simulink model "VU_NXTWay"  (Simulink 10.0)
settings: Solver=FixedStepDiscrete  StartTime=0.0  StopTime=inf  FixedStep=0.004  RelTol=1e-3
PreLoadFcn:
  | param_nxtway_gs
undefined symbols (not defined in the file): a_b, a_d, a_gc, a_gd, a_r, dst_thr, gp_max, k_f, k_i, k_phidot, k_sync, k_thetadot, pwm_gain, sound_freq, time_auto, time_start, ts1, turn_angle
libraries: lego_nxt_lib x9, simulink x1
settings Model: Creator=jpeytonj  LastModifiedBy=bhisma
settings DataIOCC: LimitDataPoints=on  SignalLoggingSaveFormat=ModelDataLogs
settings OptimizationCC: ExpressionDepthLimit=2147483647
settings DebuggingCC: SolverPrmCheckMsg=warning  SingleTaskRateTransMsg=warning  FcnCallInpInsideContextMsg=warning  StateNameClashWarn=warning
settings RTWCC: Description=Lego NXT Real-Time Target  SystemTargetFile=lrt.tlc  GenCodeOnly=on  TemplateMakefile=lrt_ecrobot.tmf
settings STFCustomTargetCC: ModelReferenceCompliant=off  GeneratePreprocessorConditionals=Disable all  MatFileLogging=on  CPPClassGenCompliant=on  SystemTargetFile=lrt.tlc
settings GRTTargetCC: ModelReferenceCompliant=off  ParMdlRefBuildCompliant=off  CompOptLevelCompliant=off  ConcurrentExecutionCompliant=off  GeneratePreprocessorConditionals=Disable all  UseToolchainInfoCompliant=off  ExtModeMexFile=noextcomm
settings CustomProperty: DataType=RTWOptions_EnumType_C__LegoMindstorms_VU-LRT_lrt_1codeGenType  Value=Integer-only
settings EnumStrPairs: String=Integer-only
settings ConfigComp: CovExternalEMLEnable=off

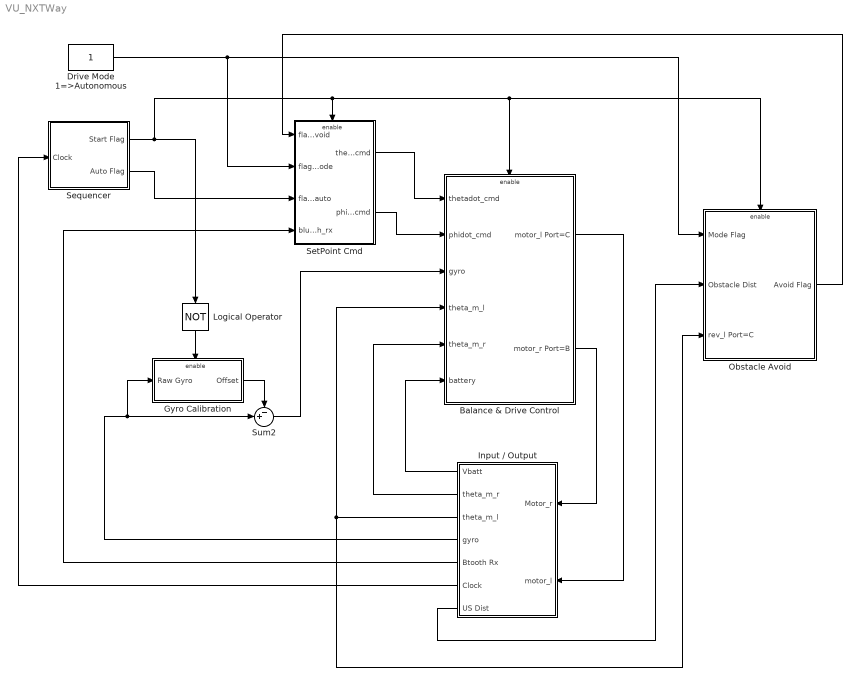
== system VU_NXTWay ==
  Balance & Drive Control : Subsystem
  Drive Mode 1=>Autonomous : Constant  OutDataTypeStr=boolean  SampleTime=-1
      settings: AttributesFormatString=DataType = %<OutDataTypeStr>
  Gyro Calibration : Subsystem  TreatAsAtomicUnit=on
  Input / Output : Subsystem
  Logical Operator : Logic  Operator=NOT  AllPortsSameDT=off  OutDataTypeStr=boolean
  Obstacle Avoid : Subsystem
  Sequencer : Subsystem
  SetPoint Cmd : Subsystem
  Sum2 : Sum  Inputs=-+|  OutDataTypeStr=Inherit: Same as first input
  wires:
  Input / Output/4(gyro) -> Gyro Calibration/1(Raw Gyro), Sum2/2
  Input / Output/1(Vbatt) -> Balance & Drive Control/6(battery)
  Logical Operator/1 -> Gyro Calibration/Enable
  Input / Output/3(theta_m_l) -> Balance & Drive Control/4(theta_m_l), Obstacle Avoid/3(rev_l Port=C)
  Input / Output/2(theta_m_r) -> Balance & Drive Control/5(theta_m_r)
  Sum2/1 -> Balance & Drive Control/3(gyro)
  Drive Mode 1=>Autonomous/1 -> Obstacle Avoid/1(Mode Flag), SetPoint Cmd/2(flag_mode)
  Balance & Drive Control/2(motor_r Port=B) -> Input / Output/1(Motor_r)
  Balance & Drive Control/1(motor_l Port=C) -> Input / Output/2(motor_l)
  Input / Output/7(US Dist) -> Obstacle Avoid/2(Obstacle Dist)
  Input / Output/6(Clock) -> Sequencer/1(Clock)
  Sequencer/1(Start Flag) -> Logical Operator/1, SetPoint Cmd/Enable, Balance & Drive Control/Enable, Obstacle Avoid/Enable
  SetPoint Cmd/1(thetadot_cmd) -> Balance & Drive Control/1(thetadot_cmd)
  SetPoint Cmd/2(phidot_cmd) -> Balance & Drive Control/2(phidot_cmd)
  Sequencer/2(Auto Flag) -> SetPoint Cmd/3(flag_auto)
  Input / Output/5(Btooth Rx) -> SetPoint Cmd/4(bluetooth_rx)
  Gyro Calibration/1(Offset) -> Sum2/1
  Obstacle Avoid/1(Avoid Flag) -> SetPoint Cmd/1(flag_avoid)

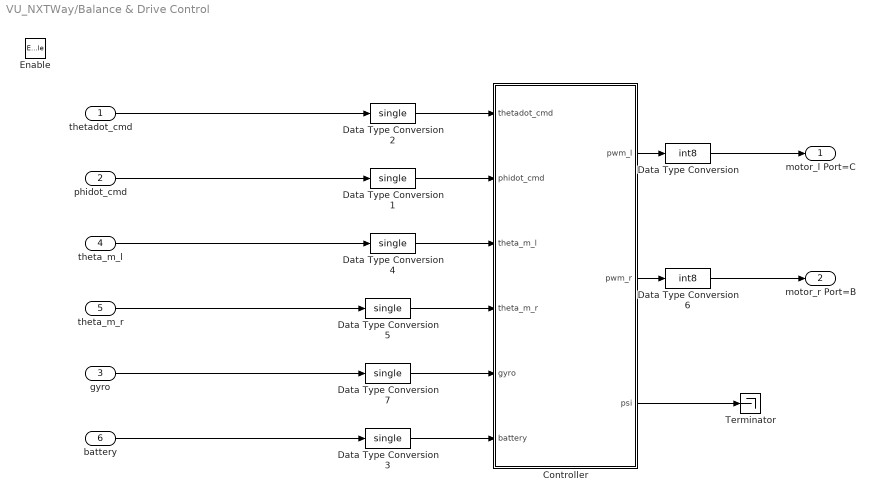
== system VU_NXTWay/Balance & Drive Control ==
  thetadot_cmd : Inport
  phidot_cmd : Inport  Port=2
  gyro : Inport  Port=3
  theta_m_l : Inport  Port=4
  theta_m_r : Inport  Port=5
  battery : Inport  Port=6
  Enable : EnablePort
  Controller : Subsystem
  Data Type Conversion : DataTypeConversion  OutDataTypeStr=int8  RndMeth=Simplest
      settings: AttributesFormatString=Round = %<RndMeth>
  Data Type Conversion{1..5,7} (6 alike) : DataTypeConversion  OutDataTypeStr=single  RndMeth=Simplest
      settings: AttributesFormatString=Round = %<RndMeth>
  Data Type Conversion6 : DataTypeConversion  OutDataTypeStr=int8  RndMeth=Simplest
      settings: AttributesFormatString=Round = %<RndMeth>
  Terminator : Terminator
  motor_l Port=C : Outport
  motor_r Port=B : Outport  Port=2
  wires:
  Data Type Conversion2/1 -> Controller/1(thetadot_cmd)
  Data Type Conversion1/1 -> Controller/2(phidot_cmd)
  Data Type Conversion6/1 -> motor_r Port=B/1
  Data Type Conversion/1 -> motor_l Port=C/1
  theta_m_r/1 -> Data Type Conversion5/1
  theta_m_l/1 -> Data Type Conversion4/1
  phidot_cmd/1 -> Data Type Conversion1/1
  thetadot_cmd/1 -> Data Type Conversion2/1
  Controller/2(pwm_r) -> Data Type Conversion6/1
  Controller/1(pwm_l) -> Data Type Conversion/1
  Data Type Conversion3/1 -> Controller/6(battery)
  battery/1 -> Data Type Conversion3/1
  Data Type Conversion5/1 -> Controller/4(theta_m_r)
  Data Type Conversion4/1 -> Controller/3(theta_m_l)
  gyro/1 -> Data Type Conversion7/1
  Data Type Conversion7/1 -> Controller/5(gyro)
  Controller/3(psi) -> Terminator/1

== system VU_NXTWay/Gyro Calibration ==
  note: Calculate gyro offset (zero point value).
  Raw Gyro : Inport
  Enable : EnablePort
  Discrete Filter : DiscreteFilter  Numerator=[1-a_gc]  Denominator=[1 -a_gc]
  Offset : Outport
  wires:
  Raw Gyro/1 -> Discrete Filter/1
  Discrete Filter/1 -> Offset/1

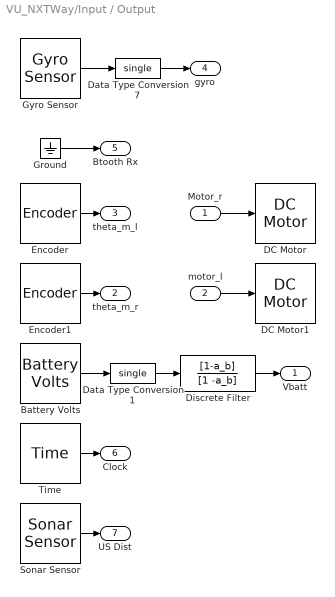
== system VU_NXTWay/Input / Output ==
  Motor_r : Inport
  motor_l : Inport  Port=2
  Battery Volts : lego_nxt_lib/Battery Volts  st=ts3
  DC Motor : lego_nxt_lib/DC Motor  port=Port C  brake=Brake
  DC Motor1 : lego_nxt_lib/DC Motor  port=Port B  brake=Brake
  Data Type Conversion1 : DataTypeConversion  OutDataTypeStr=single  RndMeth=Simplest
      settings: AttributesFormatString=Round = %<RndMeth>
  Data Type Conversion7 : DataTypeConversion  OutDataTypeStr=single  RndMeth=Simplest
      settings: AttributesFormatString=Round = %<RndMeth>
  Discrete Filter : DiscreteFilter  Numerator=[1-a_b]  Denominator=[1 -a_b]
  Encoder : lego_nxt_lib/Encoder  port=Port B  st=0.004
  Encoder1 : lego_nxt_lib/Encoder  port=Port C  st=0.004
  Ground : Ground
  Gyro Sensor : lego_nxt_lib/Gyro Sensor  port=Port 3  st=0.004
  Sonar Sensor : lego_nxt_lib/Sonar Sensor  SystemSampleTime=-1  port=Port 2  statussrc=Hide  st=0.02
  Time : lego_nxt_lib/Time  st=0.004
  Vbatt : Outport
  theta_m_r : Outport  Port=2
  theta_m_l : Outport  Port=3
  gyro : Outport  Port=4
  Btooth Rx : Outport  Port=5
  Clock : Outport  Port=6
  US Dist : Outport  Port=7
  wires:
  Gyro Sensor/1 -> Data Type Conversion7/1
  Ground/1 -> Btooth Rx/1
  Encoder/1 -> theta_m_l/1
  Encoder1/1 -> theta_m_r/1
  Battery Volts/1 -> Data Type Conversion1/1
  motor_l/1 -> DC Motor1/1
  Motor_r/1 -> DC Motor/1
  Time/1 -> Clock/1
  Sonar Sensor/1 -> US Dist/1
  Data Type Conversion7/1 -> gyro/1
  Discrete Filter/1 -> Vbatt/1
  Data Type Conversion1/1 -> Discrete Filter/1

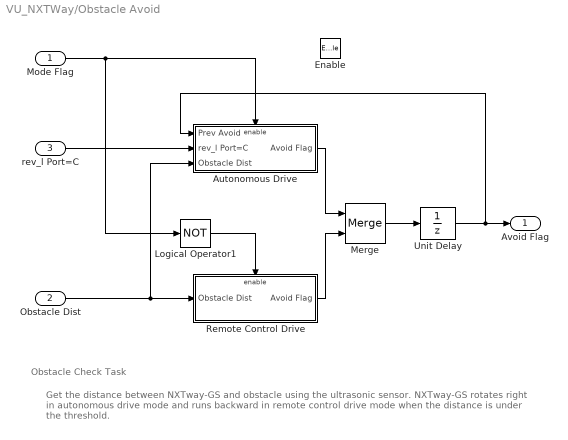
== system VU_NXTWay/Obstacle Avoid ==
  note: Get the distance between NXTway-GS and obstacle using the ultrasonic sensor.
      | NXTway-GS rotates right in autonomous drive mode and runs backward in remote
      | control drive mode when the distance is under the threshold.
  note: Obstacle Check Task
  Mode Flag : Inport
  Obstacle Dist : Inport  Port=2
  rev_l Port=C : Inport  Port=3
  Enable : EnablePort
  Autonomous Drive : Subsystem
  Logical Operator1 : Logic  Operator=NOT  AllPortsSameDT=off  OutDataTypeStr=boolean
  Merge : Merge
  Remote Control Drive : Subsystem
  Unit Delay : UnitDelay  SampleTime=-1
  Avoid Flag : Outport
  wires:
  Logical Operator1/1 -> Remote Control Drive/Enable
  Mode Flag/1 -> Logical Operator1/1, Autonomous Drive/Enable
  Obstacle Dist/1 -> Remote Control Drive/1(Obstacle Dist), Autonomous Drive/3(Obstacle Dist)
  Merge/1 -> Unit Delay/1
  Remote Control Drive/1(Avoid Flag) -> Merge/2
  Autonomous Drive/1(Avoid Flag) -> Merge/1
  rev_l Port=C/1 -> Autonomous Drive/2(rev_l Port=C)
  Unit Delay/1 -> Avoid Flag/1, Autonomous Drive/1(Prev Avoid)

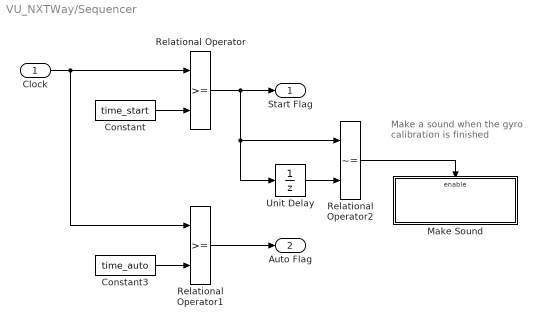
== system VU_NXTWay/Sequencer ==
  note: Make a sound when the
      | gyro calibration is finished
  Clock : Inport
  Constant : Constant  Value=time_start  OutDataTypeStr=uint32  SampleTime=0.004
      settings: AttributesFormatString=DataType = %<OutDataTypeStr>
  Constant3 : Constant  Value=time_auto  OutDataTypeStr=uint32  SampleTime=0.004
      settings: AttributesFormatString=DataType = %<OutDataTypeStr>
  Make Sound : Subsystem
  Relational Operator : RelationalOperator  OutDataTypeStr=boolean  RndMeth=Nearest
  Relational Operator1 : RelationalOperator  OutDataTypeStr=boolean  RndMeth=Nearest
  Relational Operator2 : RelationalOperator  Operator=~=  OutDataTypeStr=boolean  RndMeth=Nearest
  Unit Delay : UnitDelay  SampleTime=-1
  Start Flag : Outport
  Auto Flag : Outport  Port=2
  wires:
  Constant/1 -> Relational Operator/2
  Relational Operator/1 -> Unit Delay/1, Relational Operator2/1, Start Flag/1
  Constant3/1 -> Relational Operator1/2
  Clock/1 -> Relational Operator1/1, Relational Operator/1
  Unit Delay/1 -> Relational Operator2/2
  Relational Operator2/1 -> Make Sound/Enable
  Relational Operator1/1 -> Auto Flag/1

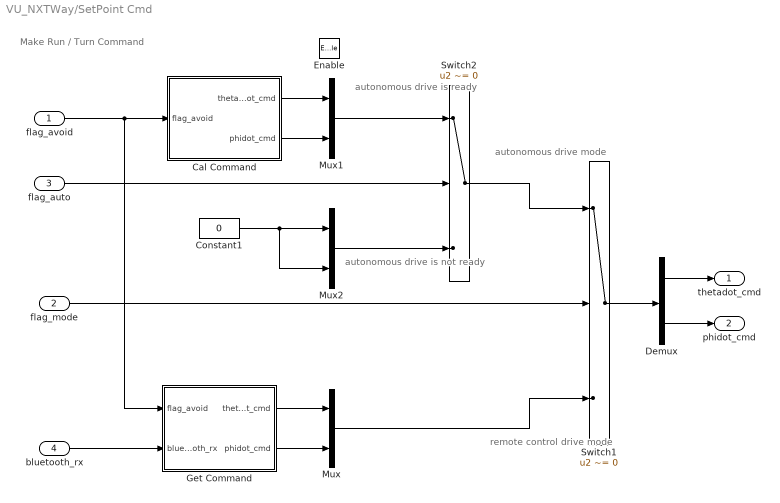
== system VU_NXTWay/SetPoint Cmd ==
  note: Make Run / Turn Command
  note: autonomous
      | drive mode
  note: remote control
      | drive mode
  note: autonomous
      | drive is ready
  note: autonomous
      | drive is not ready
  flag_avoid : Inport
  flag_mode : Inport  Port=2
  flag_auto : Inport  Port=3
  bluetooth_rx : Inport  Port=4
  Enable : EnablePort
  Cal Command : Subsystem
  Constant1 : Constant  Value=0  VectorParams1D=off  OutDataTypeStr=int8  SampleTime=0.004
      settings: AttributesFormatString=DataType = %<OutDataTypeStr>
  Demux : Demux  Outputs=2
  Get Command : Subsystem
  Mux : Mux  Inputs=2
  Mux1 : Mux  Inputs=2
  Mux2 : Mux  Inputs=2
  Switch1 : Switch  Criteria=u2 ~= 0
  Switch2 : Switch  Criteria=u2 ~= 0
  thetadot_cmd : Outport
  phidot_cmd : Outport  Port=2
  wires:
  bluetooth_rx/1 -> Get Command/2(bluetooth_rx)
  flag_mode/1 -> Switch1/2
  Get Command/1(thetadot_cmd) -> Mux/1
  Get Command/2(phidot_cmd) -> Mux/2
  Demux/2 -> phidot_cmd/1
  Cal Command/1(thetadot_cmd) -> Mux1/1
  Cal Command/2(phidot_cmd) -> Mux1/2
  Mux/1 -> Switch1/3
  flag_auto/1 -> Switch2/2
  Mux1/1 -> Switch2/1
  Constant1/1 -> Mux2/1, Mux2/2
  Mux2/1 -> Switch2/3
  Switch2/1 -> Switch1/1
  flag_avoid/1 -> Cal Command/1(flag_avoid), Get Command/1(flag_avoid)
  Switch1/1 -> Demux/1
  Demux/1 -> thetadot_cmd/1

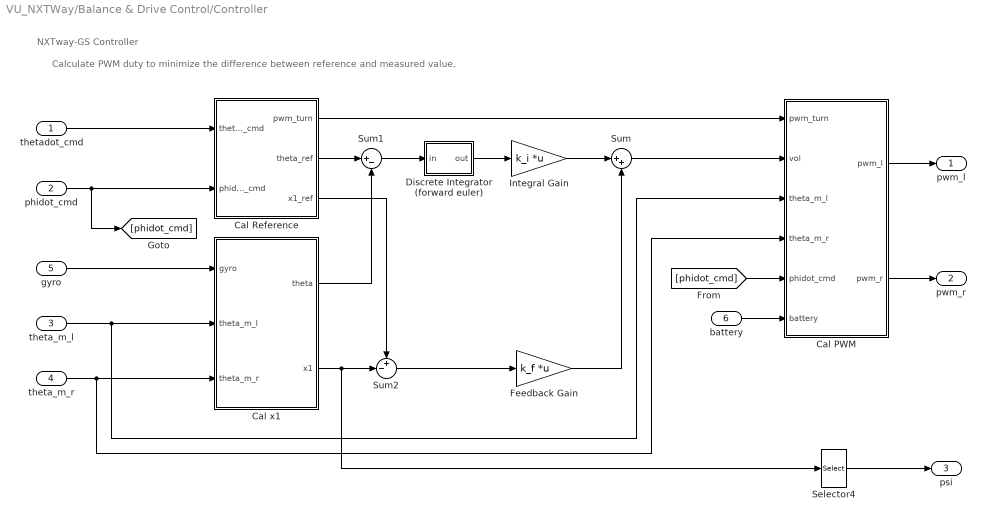
== system VU_NXTWay/Balance & Drive Control/Controller ==
  note: Calculate PWM duty to minimize the difference between reference and measured value.
  note: NXTway-GS Controller
  thetadot_cmd : Inport
  phidot_cmd : Inport  Port=2
  theta_m_l : Inport  Port=3
  theta_m_r : Inport  Port=4
  gyro : Inport  Port=5
  battery : Inport  Port=6
  Cal PWM : Subsystem
  Cal Reference : Subsystem
  Cal x1 : Subsystem
  Discrete Integrator (forward euler) : Subsystem
  Feedback Gain : Gain  Gain=k_f  Multiplication=Matrix(K*u)  OutDataTypeStr=Inherit: Same as input  ParamDataTypeStr=Inherit: Same as input
  Integral Gain : Gain  Gain=k_i  Multiplication=Matrix(K*u)  OutDataTypeStr=Inherit: Same as input  ParamDataTypeStr=Inherit: Same as input
  Selector4 : Selector  InputPortWidth=4  IndexOptions=Index vector (dialog)  Indices=2  OutputSizes=1
  Sum : Sum  Inputs=|++  OutDataTypeStr=Inherit: Same as first input
  Sum1 : Sum  Inputs=|+-  OutDataTypeStr=Inherit: Same as first input
  Sum2 : Sum  Inputs=+-|  OutDataTypeStr=Inherit: Same as first input
  pwm_l : Outport
  pwm_r : Outport  Port=2
  psi : Outport  Port=3
  wires:
  [phidot_cmd] -> Cal PWM/5(phidot_cmd)
  Selector4/1 -> psi/1
  Cal Reference/3(x1_ref) -> Sum2/1
  Sum2/1 -> Feedback Gain/1
  Cal x1/2(x1) -> Selector4/1, Sum2/2
  Integral Gain/1 -> Sum/1
  Discrete Integrator (forward euler)/1(out) -> Integral Gain/1
  Sum1/1 -> Discrete Integrator (forward euler)/1(in)
  Cal x1/1(theta) -> Sum1/2
  Cal Reference/2(theta_ref) -> Sum1/1
  Feedback Gain/1 -> Sum/2
  theta_m_r/1 -> Cal PWM/4(theta_m_r), Cal x1/3(theta_m_r)
  battery/1 -> Cal PWM/6(battery)
  Sum/1 -> Cal PWM/2(vol)
  phidot_cmd/1 -> [phidot_cmd], Cal Reference/2(phidot_cmd)
  thetadot_cmd/1 -> Cal Reference/1(thetadot_cmd)
  Cal Reference/1(pwm_turn) -> Cal PWM/1(pwm_turn)
  Cal PWM/1(pwm_l) -> pwm_l/1
  Cal PWM/2(pwm_r) -> pwm_r/1
  theta_m_l/1 -> Cal PWM/3(theta_m_l), Cal x1/2(theta_m_l)
  gyro/1 -> Cal x1/1(gyro)

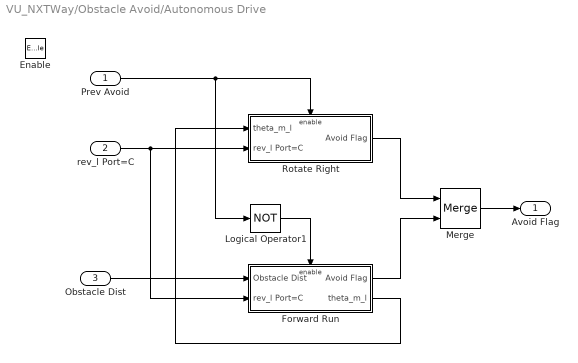
== system VU_NXTWay/Obstacle Avoid/Autonomous Drive ==
  Prev Avoid : Inport
  rev_l Port=C : Inport  Port=2
  Obstacle Dist : Inport  Port=3
  Enable : EnablePort
  Forward Run : Subsystem
  Logical Operator1 : Logic  Operator=NOT  AllPortsSameDT=off  OutDataTypeStr=boolean
  Merge : Merge
  Rotate Right : Subsystem
  Avoid Flag : Outport
  wires:
  Forward Run/2(theta_m_l) -> Rotate Right/1(theta_m_l)
  Logical Operator1/1 -> Forward Run/Enable
  Forward Run/1(Avoid Flag) -> Merge/2
  Merge/1 -> Avoid Flag/1
  Rotate Right/1(Avoid Flag) -> Merge/1
  rev_l Port=C/1 -> Rotate Right/2(rev_l Port=C), Forward Run/2(rev_l Port=C)
  Obstacle Dist/1 -> Forward Run/1(Obstacle Dist)
  Prev Avoid/1 -> Rotate Right/Enable, Logical Operator1/1

== system VU_NXTWay/Obstacle Avoid/Remote Control Drive ==
  Obstacle Dist : Inport
  Enable : EnablePort
  Constant : Constant  Value=dst_thr  OutDataTypeStr=int32  SampleTime=0.004
      settings: AttributesFormatString=DataType = %<OutDataTypeStr>
  Relational Operator : RelationalOperator  Operator=<=  OutDataTypeStr=boolean  RndMeth=Nearest
  Avoid Flag : Outport
  wires:
  Obstacle Dist/1 -> Relational Operator/1
  Relational Operator/1 -> Avoid Flag/1
  Constant/1 -> Relational Operator/2

== system VU_NXTWay/Sequencer/Make Sound ==
  Enable : EnablePort
  Constant : Constant  Value=sound_freq  OutDataTypeStr=uint32  SampleTime=0.2
      settings: AttributesFormatString=DataType = %<OutDataTypeStr>
  Sound Tone : lego_nxt_lib/Sound Tone  SystemSampleTime=-1  freqsrc=External  freq=0  volsrc=Internal  vol=20
  wires:
  Constant/1 -> Sound Tone/1

== system VU_NXTWay/SetPoint Cmd/Cal Command ==
  note: NXTway-GS rotates right when it is avoiding obstacle.
  flag_avoid : Inport
  Constant : Constant  Value=gp_max  VectorParams1D=off  OutDataTypeStr=int8  SampleTime=0.004
      settings: AttributesFormatString=DataType = %<OutDataTypeStr>
  Constant1 : Constant  Value=0  VectorParams1D=off  OutDataTypeStr=int8  SampleTime=0.004
      settings: AttributesFormatString=DataType = %<OutDataTypeStr>
  Constant2 : Constant  Value=0  VectorParams1D=off  OutDataTypeStr=int8  SampleTime=0.004
      settings: AttributesFormatString=DataType = %<OutDataTypeStr>
  Constant3 : Constant  Value=gp_max  VectorParams1D=off  OutDataTypeStr=int8  SampleTime=0.004
      settings: AttributesFormatString=DataType = %<OutDataTypeStr>
  Switch : Switch  Criteria=u2 ~= 0
  Switch2 : Switch  Criteria=u2 ~= 0
  thetadot_cmd : Outport
  phidot_cmd : Outport  Port=2
  wires:
  flag_avoid/1 -> Switch2/2, Switch/2  "flag_turn"
  Constant1/1 -> Switch/1
  Constant/1 -> Switch/3
  Constant3/1 -> Switch2/1
  Constant2/1 -> Switch2/3
  Switch/1 -> thetadot_cmd/1
  Switch2/1 -> phidot_cmd/1

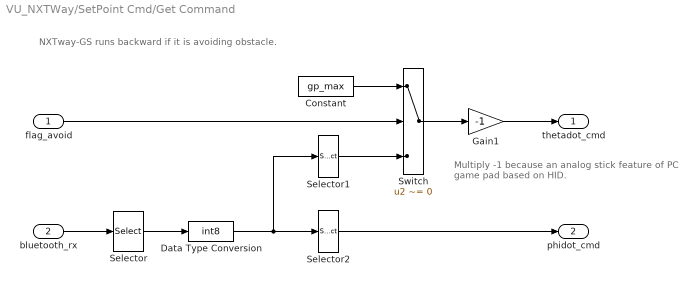
== system VU_NXTWay/SetPoint Cmd/Get Command ==
  note: Multiply -1 because an analog stick
      | feature of PC game pad based on HID.
  note: NXTway-GS runs backward if it is avoiding obstacle.
  flag_avoid : Inport
  bluetooth_rx : Inport  Port=2
  Constant : Constant  Value=gp_max  VectorParams1D=off  OutDataTypeStr=int8  SampleTime=0.004
      settings: AttributesFormatString=DataType = %<OutDataTypeStr>
  Data Type Conversion : DataTypeConversion  OutDataTypeStr=int8  RndMeth=Simplest
      settings: AttributesFormatString=Round = %<RndMeth>
  Gain1 : Gain  Gain=-1  OutDataTypeStr=Inherit: Same as input  ParamDataTypeStr=Inherit: Same as input
  Selector : Selector  InputPortWidth=32  IndexOptions=Index vector (dialog)  Indices=[1 2]  OutputSizes=1
      settings: AttributesFormatString=Indices = %<Indices>
  Selector1 : Selector  InputPortWidth=2  IndexOptions=Index vector (dialog)  Indices=1  OutputSizes=1
  Selector2 : Selector  InputPortWidth=2  IndexOptions=Index vector (dialog)  Indices=2  OutputSizes=1
  Switch : Switch  Criteria=u2 ~= 0
  thetadot_cmd : Outport
  phidot_cmd : Outport  Port=2
  wires:
  Selector/1 -> Data Type Conversion/1
  Data Type Conversion/1 -> Selector2/1, Selector1/1
  Selector1/1 -> Switch/3
  bluetooth_rx/1 -> Selector/1
  Selector2/1 -> phidot_cmd/1
  Switch/1 -> Gain1/1
  Constant/1 -> Switch/1
  Gain1/1 -> thetadot_cmd/1
  flag_avoid/1 -> Switch/2

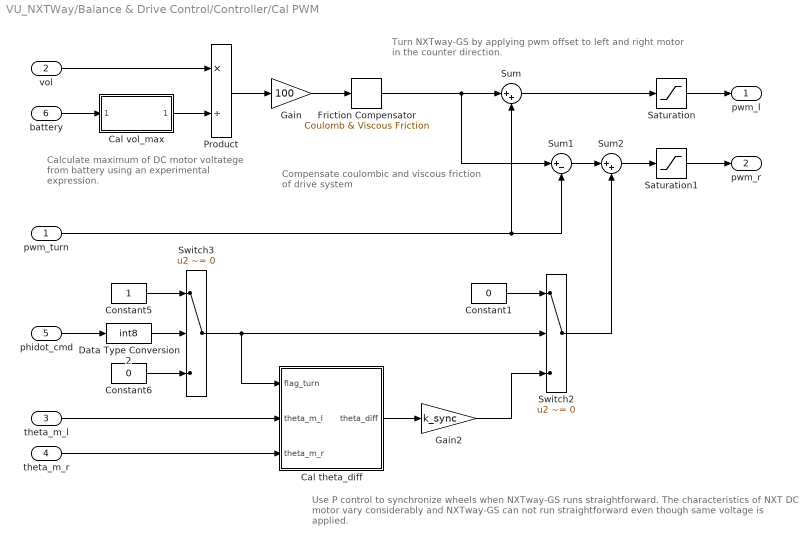
== system VU_NXTWay/Balance & Drive Control/Controller/Cal PWM ==
  note: Compensate coulombic and
      | viscous friction of drive system
  note: Turn NXTway-GS by applying pwm offset
      | to left and right motor in the counter direction.
  note: Use P control to synchronize wheels when NXTway-GS runs straightforward.
      | The characteristics of NXT DC motor vary considerably and NXTway-GS can not
      | run straightforward even though same voltage is applied.
  note: Calculate maximum of DC motor
      | voltatege from battery using an
      | experimental expression.
  pwm_turn : Inport
  vol : Inport  Port=2
  theta_m_l : Inport  Port=3
  theta_m_r : Inport  Port=4
  phidot_cmd : Inport  Port=5
  battery : Inport  Port=6
  Cal theta_diff : Subsystem
  Cal vol_max : Subsystem
  Constant1 : Constant  Value=0  OutDataTypeStr=single  SampleTime=-1
      settings: AttributesFormatString=DataType = %<OutDataTypeStr>
  Constant5 : Constant  OutDataTypeStr=boolean  SampleTime=-1
      settings: AttributesFormatString=DataType = %<OutDataTypeStr>
  Constant6 : Constant  Value=0  OutDataTypeStr=boolean  SampleTime=-1
      settings: AttributesFormatString=DataType = %<OutDataTypeStr>
  Data Type Conversion2 : DataTypeConversion  OutDataTypeStr=int8  RndMeth=Simplest
      settings: AttributesFormatString=Round = %<RndMeth>
  Friction Compensator : simulink/Discontinuities/Coulomb & Viscous Friction  SystemSampleTime=-1  offset=pwm_offset  gain=pwm_gain
      settings: AttributesFormatString=gain = %<gain>\noffset = %<offset>  SourceProductName=Simulink
  Gain : Gain  Gain=100  OutDataTypeStr=Inherit: Same as input  ParamDataTypeStr=Inherit: Same as input
  Gain2 : Gain  Gain=k_sync  OutDataTypeStr=Inherit: Same as input  ParamDataTypeStr=Inherit: Same as input
  Product : Product  Inputs=*/  RndMeth=Simplest  OutDataTypeStr=Inherit: Same as first input
  Saturation : Saturate  UpperLimit=100  LowerLimit=-100
      settings: AttributesFormatString=max = %<UpperLimit>\nmin = %<LowerLimit>
  Saturation1 : Saturate  UpperLimit=100  LowerLimit=-100
      settings: AttributesFormatString=max = %<UpperLimit>\nmin = %<LowerLimit>
  Sum : Sum  Inputs=|++  OutDataTypeStr=Inherit: Same as first input
  Sum1 : Sum  Inputs=|+-  OutDataTypeStr=Inherit: Same as first input
  Sum2 : Sum  Inputs=|++  OutDataTypeStr=Inherit: Same as first input
  Switch2 : Switch  Criteria=u2 ~= 0
  Switch3 : Switch  Criteria=u2 ~= 0
  pwm_l : Outport
  pwm_r : Outport  Port=2
  wires:
  Data Type Conversion2/1 -> Switch3/2
  phidot_cmd/1 -> Data Type Conversion2/1
  Constant6/1 -> Switch3/3
  Constant5/1 -> Switch3/1
  theta_m_r/1 -> Cal theta_diff/3(theta_m_r)
  theta_m_l/1 -> Cal theta_diff/2(theta_m_l)
  Friction Compensator/1 -> Sum/1, Sum1/1
  Sum2/1 -> Saturation1/1
  Sum1/1 -> Sum2/1
  Cal vol_max/1(vol_max) -> Product/2
  battery/1 -> Cal vol_max/1(battery)
  Gain2/1 -> Switch2/3
  Constant1/1 -> Switch2/1
  Switch3/1 -> Cal theta_diff/1(flag_turn), Switch2/2
  Cal theta_diff/1(theta_diff) -> Gain2/1
  Product/1 -> Gain/1
  vol/1 -> Product/1
  Saturation/1 -> pwm_l/1
  Saturation1/1 -> pwm_r/1
  Gain/1 -> Friction Compensator/1
  pwm_turn/1 -> Sum1/2, Sum/2
  Sum/1 -> Saturation/1
  Switch2/1 -> Sum2/2

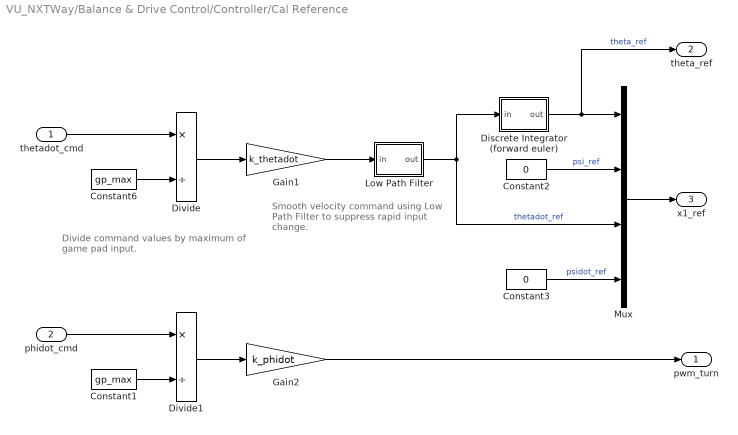
== system VU_NXTWay/Balance & Drive Control/Controller/Cal Reference ==
  note: Smooth velocity command
      | using Low Path Filter to
      | suppress rapid input change.
  note: Divide command values by
      | maximum of game pad input.
  thetadot_cmd : Inport
  phidot_cmd : Inport  Port=2
  Constant1 : Constant  Value=gp_max  VectorParams1D=off  OutDataTypeStr=int8  SampleTime=-1
      settings: AttributesFormatString=DataType = %<OutDataTypeStr>
  Constant2 : Constant  Value=0  VectorParams1D=off  OutDataTypeStr=single  SampleTime=-1
      settings: AttributesFormatString=DataType = %<OutDataTypeStr>
  Constant3 : Constant  Value=0  VectorParams1D=off  OutDataTypeStr=single  SampleTime=-1
      settings: AttributesFormatString=DataType = %<OutDataTypeStr>
  Constant6 : Constant  Value=gp_max  VectorParams1D=off  OutDataTypeStr=int8  SampleTime=-1
      settings: AttributesFormatString=DataType = %<OutDataTypeStr>
  Discrete Integrator (forward euler) : Subsystem
  Divide : Product  Inputs=*/  RndMeth=Simplest  OutDataTypeStr=Inherit: Same as first input
  Divide1 : Product  Inputs=*/  RndMeth=Simplest  OutDataTypeStr=Inherit: Same as first input
  Gain1 : Gain  Gain=k_thetadot  OutDataTypeStr=Inherit: Same as input  ParamDataTypeStr=Inherit: Same as input
  Gain2 : Gain  Gain=k_phidot  OutDataTypeStr=Inherit: Same as input  ParamDataTypeStr=Inherit: Same as input
  Low Path Filter : Subsystem
  Mux : Mux
  pwm_turn : Outport
  theta_ref : Outport  Port=2
  x1_ref : Outport  Port=3
  wires:
  Constant6/1 -> Divide/2
  Low Path Filter/1(out) -> Mux/3, Discrete Integrator (forward euler)/1(in)  "thetadot_ref"
  Constant3/1 -> Mux/4  "psidot_ref"
  Constant2/1 -> Mux/2  "psi_ref"
  Discrete Integrator (forward euler)/1(out) -> Mux/1, theta_ref/1  "theta_ref"
  Mux/1 -> x1_ref/1
  Divide1/1 -> Gain2/1
  Constant1/1 -> Divide1/2
  Gain2/1 -> pwm_turn/1
  Divide/1 -> Gain1/1
  thetadot_cmd/1 -> Divide/1
  Gain1/1 -> Low Path Filter/1(in)
  phidot_cmd/1 -> Divide1/1

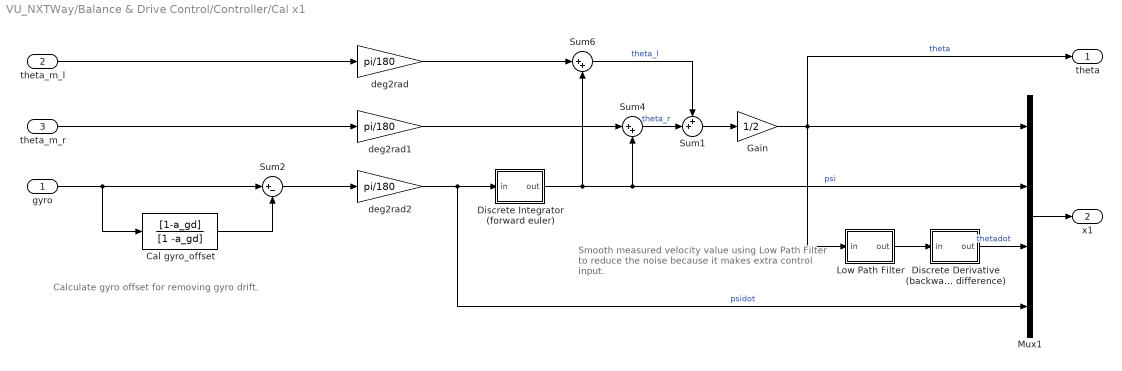
== system VU_NXTWay/Balance & Drive Control/Controller/Cal x1 ==
  note: Smooth measured velocity value using
      | Low Path Filter to reduce the noise
      | because it makes extra control input.
  note: Calculate gyro offset for removing gyro drift.
  gyro : Inport
  theta_m_l : Inport  Port=2
  theta_m_r : Inport  Port=3
  Cal gyro_offset : DiscreteFilter  Numerator=[1-a_gd]  Denominator=[1 -a_gd]
  Discrete Derivative (backward difference) : Subsystem
  Discrete Integrator (forward euler) : Subsystem
  Gain : Gain  Gain=1/2  OutDataTypeStr=Inherit: Same as input  ParamDataTypeStr=Inherit: Same as input
  Low Path Filter : Subsystem
  Mux1 : Mux
  Sum1 : Sum  Inputs=++|  OutDataTypeStr=Inherit: Same as first input
  Sum2 : Sum  Inputs=|+-  OutDataTypeStr=Inherit: Same as first input
  Sum4 : Sum  Inputs=|++  OutDataTypeStr=Inherit: Same as first input
  Sum6 : Sum  Inputs=|++  OutDataTypeStr=Inherit: Same as first input
  deg2rad : Gain  Gain=pi/180  OutDataTypeStr=Inherit: Same as input  ParamDataTypeStr=Inherit: Same as input
  deg2rad1 : Gain  Gain=pi/180  OutDataTypeStr=Inherit: Same as input  ParamDataTypeStr=Inherit: Same as input
  deg2rad2 : Gain  Gain=pi/180  OutDataTypeStr=Inherit: Same as input  ParamDataTypeStr=Inherit: Same as input
  theta : Outport
  x1 : Outport  Port=2
  wires:
  Gain/1 -> Low Path Filter/1(in), Mux1/1, theta/1  "theta"
  Low Path Filter/1(out) -> Discrete Derivative (backward difference)/1(in)
  deg2rad2/1 -> Mux1/4, Discrete Integrator (forward euler)/1(in)  "psidot"
  Sum1/1 -> Gain/1
  Sum4/1 -> Sum1/2  "theta_r"
  Sum6/1 -> Sum1/1  "theta_l"
  Discrete Derivative (backward difference)/1(out) -> Mux1/3  "thetadot"
  theta_m_r/1 -> deg2rad1/1
  theta_m_l/1 -> deg2rad/1
  deg2rad/1 -> Sum6/1
  Discrete Integrator (forward euler)/1(out) -> Mux1/2, Sum4/2, Sum6/2  "psi"
  Mux1/1 -> x1/1
  deg2rad1/1 -> Sum4/1
  Sum2/1 -> deg2rad2/1
  Cal gyro_offset/1 -> Sum2/2
  gyro/1 -> Sum2/1, Cal gyro_offset/1

== system VU_NXTWay/Balance & Drive Control/Controller/Discrete Integrator (forward euler) ==
  in : Inport
  Gain : Gain  Gain=ts1  OutDataTypeStr=Inherit: Same as input  ParamDataTypeStr=Inherit: Same as input
  Sum : Sum  Inputs=|++  OutDataTypeStr=Inherit: Same as first input
  Unit Delay : UnitDelay  SampleTime=-1
  out : Outport
  wires:
  in/1 -> Gain/1
  Sum/1 -> Unit Delay/1
  Gain/1 -> Sum/1
  Unit Delay/1 -> out/1, Sum/2

== system VU_NXTWay/Obstacle Avoid/Autonomous Drive/Forward Run ==
  note: Set flag_avoid and store left motor revolution angle.
  Obstacle Dist : Inport
  rev_l Port=C : Inport  Port=2
  Enable : EnablePort
  Constant : Constant  Value=dst_thr  OutDataTypeStr=int32  SampleTime=0.004
      settings: AttributesFormatString=DataType = %<OutDataTypeStr>
  Relational Operator : RelationalOperator  Operator=<=  OutDataTypeStr=boolean  RndMeth=Nearest
  Avoid Flag : Outport
  theta_m_l : Outport  Port=2
  wires:
  Relational Operator/1 -> Avoid Flag/1
  Constant/1 -> Relational Operator/2
  Obstacle Dist/1 -> Relational Operator/1
  rev_l Port=C/1 -> theta_m_l/1

== system VU_NXTWay/Obstacle Avoid/Autonomous Drive/Rotate Right ==
  note: NXTway-GS rotates right by turn_angle [deg].
  theta_m_l : Inport
  rev_l Port=C : Inport  Port=2
  Enable : EnablePort
  Constant1 : Constant  Value=turn_angle  OutDataTypeStr=int32  SampleTime=0.004
      settings: AttributesFormatString=DataType = %<OutDataTypeStr>
  Relational Operator1 : RelationalOperator  Operator=<=  OutDataTypeStr=boolean  RndMeth=Nearest
  Sum1 : Sum  Inputs=|+-  OutDataTypeStr=Inherit: Same as first input
  Avoid Flag : Outport
  wires:
  Relational Operator1/1 -> Avoid Flag/1
  theta_m_l/1 -> Sum1/2
  Sum1/1 -> Relational Operator1/1
  rev_l Port=C/1 -> Sum1/1
  Constant1/1 -> Relational Operator1/2

== system VU_NXTWay/Balance & Drive Control/Controller/Cal PWM/Cal theta_diff ==
  note: Save the difference between
      | left and right motor revolution angle
  note: Detect turn -> straight run change
  flag_turn : Inport
  theta_m_l : Inport  Port=2
  theta_m_r : Inport  Port=3
  Detect Flag Falling : Subsystem
  Set theta_offset : Subsystem
  Sum1 : Sum  Inputs=|+-  OutDataTypeStr=Inherit: Same as first input
  Sum5 : Sum  Inputs=|-+  OutDataTypeStr=Inherit: Same as first input
  theta_diff : Outport
  wires:
  Set theta_offset/1(theta_offset) -> Sum5/1
  theta_m_r/1 -> Sum1/2
  theta_m_l/1 -> Sum1/1
  Sum1/1 -> Sum5/2, Set theta_offset/1(theta_diff)
  Detect Flag Falling/1(falling) -> Set theta_offset/Enable
  Sum5/1 -> theta_diff/1
  flag_turn/1 -> Detect Flag Falling/1(flag)

== system VU_NXTWay/Balance & Drive Control/Controller/Cal PWM/Cal vol_max ==
  battery : Inport
  Constant : Constant  Value=0.625  OutDataTypeStr=single  SampleTime=-1
      settings: AttributesFormatString=DataType = %<OutDataTypeStr>
  Gain3 : Gain  Gain=0.001089  OutDataTypeStr=Inherit: Same as input  ParamDataTypeStr=Inherit: Same as input
  Sum2 : Sum  Inputs=|+-  OutDataTypeStr=Inherit: Same as first input
  vol_max : Outport
  wires:
  battery/1 -> Gain3/1
  Gain3/1 -> Sum2/1
  Sum2/1 -> vol_max/1
  Constant/1 -> Sum2/2

== system VU_NXTWay/Balance & Drive Control/Controller/Cal Reference/Discrete Integrator (forward euler) ==
  in : Inport
  Gain : Gain  Gain=ts1  OutDataTypeStr=Inherit: Same as input  ParamDataTypeStr=Inherit: Same as input
  Sum : Sum  Inputs=|++  OutDataTypeStr=Inherit: Same as first input
  Unit Delay : UnitDelay  SampleTime=-1
  out : Outport
  wires:
  in/1 -> Gain/1
  Sum/1 -> Unit Delay/1
  Gain/1 -> Sum/1
  Unit Delay/1 -> out/1, Sum/2

== system VU_NXTWay/Balance & Drive Control/Controller/Cal Reference/Low Path Filter ==
  note: Low Path Filter Function
      |               1-a_r
      |          ----------------
      |          1-a_r*z^(-1)
  in : Inport
  Gain2 : Gain  Gain=a_r  OutDataTypeStr=Inherit: Same as input  ParamDataTypeStr=Inherit: Same as input
  Gain3 : Gain  Gain=1-a_r  OutDataTypeStr=Inherit: Same as input  ParamDataTypeStr=Inherit: Same as input
  Sum : Sum  Inputs=|++  OutDataTypeStr=Inherit: Same as first input
  Unit Delay : UnitDelay  SampleTime=-1
  out : Outport
  wires:
  in/1 -> Gain3/1
  Gain3/1 -> Sum/1
  Gain2/1 -> Sum/2
  Unit Delay/1 -> Gain2/1
  Sum/1 -> out/1, Unit Delay/1

== system VU_NXTWay/Balance & Drive Control/Controller/Cal x1/Discrete Derivative (backward difference) ==
  in : Inport
  Gain : Gain  Gain=1/ts1  OutDataTypeStr=Inherit: Same as input  ParamDataTypeStr=Inherit: Same as input
  Sum : Sum  Inputs=|+-  OutDataTypeStr=Inherit: Same as first input
  Unit Delay : UnitDelay  SampleTime=-1
  out : Outport
  wires:
  Gain/1 -> out/1
  in/1 -> Sum/1, Unit Delay/1
  Unit Delay/1 -> Sum/2
  Sum/1 -> Gain/1

== system VU_NXTWay/Balance & Drive Control/Controller/Cal x1/Discrete Integrator (forward euler) ==
  in : Inport
  Gain : Gain  Gain=ts1  OutDataTypeStr=Inherit: Same as input  ParamDataTypeStr=Inherit: Same as input
  Sum : Sum  Inputs=|++  OutDataTypeStr=Inherit: Same as first input
  Unit Delay : UnitDelay  SampleTime=-1
  out : Outport
  wires:
  Unit Delay/1 -> Sum/2, out/1
  Gain/1 -> Sum/1
  Sum/1 -> Unit Delay/1
  in/1 -> Gain/1

== system VU_NXTWay/Balance & Drive Control/Controller/Cal x1/Low Path Filter ==
  note: Low Path Filter Function
      |               1-a_d
      |          ----------------
      |          1-a_d*z^(-1)
  in : Inport
  Gain2 : Gain  Gain=a_d  OutDataTypeStr=Inherit: Same as input  ParamDataTypeStr=Inherit: Same as input
  Gain3 : Gain  Gain=1-a_d  OutDataTypeStr=Inherit: Same as input  ParamDataTypeStr=Inherit: Same as input
  Sum : Sum  Inputs=|++  OutDataTypeStr=Inherit: Same as first input
  Unit Delay : UnitDelay  SampleTime=-1
  out : Outport
  wires:
  in/1 -> Gain3/1
  Gain3/1 -> Sum/1
  Gain2/1 -> Sum/2
  Unit Delay/1 -> Gain2/1
  Sum/1 -> out/1, Unit Delay/1

== system VU_NXTWay/Balance & Drive Control/Controller/Cal PWM/Cal theta_diff/Detect Flag Falling ==
  flag : Inport
  Constant : Constant  Value=0  VectorParams1D=off  OutDataTypeStr=boolean  SampleTime=-1
      settings: AttributesFormatString=DataType = %<OutDataTypeStr>
  Constant1 : Constant  VectorParams1D=off  OutDataTypeStr=boolean  SampleTime=-1
      settings: AttributesFormatString=DataType = %<OutDataTypeStr>
  Logical Operator : Logic  AllPortsSameDT=off  OutDataTypeStr=boolean
  Relational Operator : RelationalOperator  Operator===  OutDataTypeStr=boolean  RndMeth=Nearest
  Relational Operator1 : RelationalOperator  Operator===  OutDataTypeStr=boolean  RndMeth=Nearest
  Unit Delay : UnitDelay  SampleTime=-1
  falling : Outport
  wires:
  Logical Operator/1 -> falling/1
  Relational Operator1/1 -> Logical Operator/2
  Relational Operator/1 -> Logical Operator/1
  Constant1/1 -> Relational Operator1/2
  Unit Delay/1 -> Relational Operator1/1
  Constant/1 -> Relational Operator/2
  flag/1 -> Relational Operator/1, Unit Delay/1

== system VU_NXTWay/Balance & Drive Control/Controller/Cal PWM/Cal theta_diff/Set theta_offset ==
  theta_diff : Inport
  Enable : EnablePort
  theta_offset : Outport
  wires:
  theta_diff/1 -> theta_offset/1
